simulink model "ACC_CTG_Multi_Simul"  (R2022b)
settings: Solver=VariableStepAuto  StartTime=0.0  StopTime=t_end  FixedStep=0.001  RelTol=1e-3
values from neighbouring files (symbols this model uses):
  Af = 4    [ABS_Simul_Initialize.m]    (also in ACC_CTG_Multi_Simul_Initialize.m; ACC_Space_Single_Simul_Initialize.m; ACC_Space_multi_Simul_Initialize.m; CruiseControl_Initialize.m)
  Cd = 0.3    [ABS_Simul_Initialize.m]    (also in ACC_CTG_Multi_Simul_Initialize.m; ACC_Space_Single_Simul_Initialize.m; ACC_Space_multi_Simul_Initialize.m; CruiseControl_Initialize.m)
  delta_12_0 = 600    [ACC_CTG_Multi_Simul_Initialize.m]    (also in ACC_Space_multi_Simul_Initialize.m = 550)
  delta_h1_0 = 600    [ACC_CTG_Multi_Simul_Initialize.m]    (also in ACC_Space_multi_Simul_Initialize.m = 550)
  g = 9.81    [ABS_Simul_Initialize.m]    (also in ACC_CTG_Multi_Simul_Initialize.m; ACC_Space_Single_Simul_Initialize.m; ACC_Space_multi_Simul_Initialize.m; CruiseControl_Initialize.m)
  h = 0.65    [ABS_Simul_Initialize.m]    (also in ACC_CTG_Multi_Simul_Initialize.m = 10; ACC_Space_Single_Simul_Initialize.m; ACC_Space_multi_Simul_Initialize.m; CruiseControl_Initialize.m)
  Ki_Cruise = 0.1    [ACC_CTG_Multi_Simul_Initialize.m]    (also in ACC_Space_Single_Simul_Initialize.m; ACC_Space_multi_Simul_Initialize.m)
  Kp_Cruise = 1    [ACC_CTG_Multi_Simul_Initialize.m]    (also in ACC_Space_Single_Simul_Initialize.m; ACC_Space_multi_Simul_Initialize.m)
  L_ACC = 500    [ACC_CTG_Multi_Simul_Initialize.m]    (also in ACC_Space_Single_Simul_Initialize.m; ACC_Space_multi_Simul_Initialize.m)
  lr = 1.8    [ABS_Simul_Initialize.m]    (also in ACC_CTG_Multi_Simul_Initialize.m; ACC_Space_Single_Simul_Initialize.m; ACC_Space_multi_Simul_Initialize.m; CruiseControl_Initialize.m)
  m = 1500    [ABS_Simul_Initialize.m]    (also in ACC_CTG_Multi_Simul_Initialize.m; ACC_Space_Single_Simul_Initialize.m; ACC_Space_multi_Simul_Initialize.m; CruiseControl_Initialize.m)
  ramda = 1    [ACC_CTG_Multi_Simul_Initialize.m]
  rho = 1.225    [ABS_Simul_Initialize.m]    (also in ACC_CTG_Multi_Simul_Initialize.m; ACC_Space_Single_Simul_Initialize.m; ACC_Space_multi_Simul_Initialize.m; CruiseControl_Initialize.m)
  tau = 0.5    [ACC_CTG_Multi_Simul_Initialize.m]    (also in ACC_Space_multi_Simul_Initialize.m)
  V_desire = 120    [ACC_CTG_Multi_Simul_Initialize.m]    (also in ACC_Space_Single_Simul_Initialize.m; ACC_Space_multi_Simul_Initialize.m; CruiseControl_Initialize.m = 100)
  xdot1_0 = 80    [ACC_CTG_Multi_Simul_Initialize.m]    (also in ACC_Space_multi_Simul_Initialize.m)
  xdot2_0 = 80    [ACC_CTG_Multi_Simul_Initialize.m]    (also in ACC_Space_multi_Simul_Initialize.m)
libraries: autolibshared x2, simulink x2
settings Model: Creator=lego0  LastModifiedBy=lego0

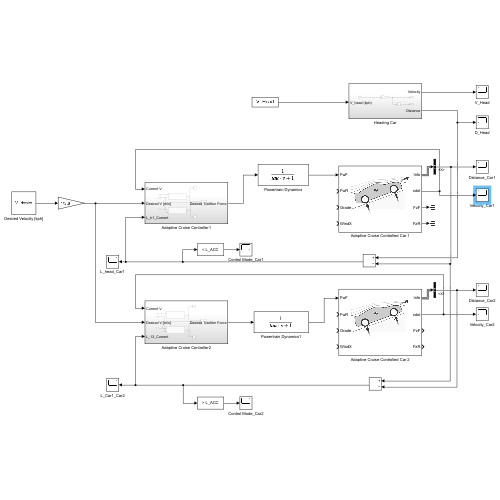
[thumbnail: Simulink's stored preview of the top-level diagram]
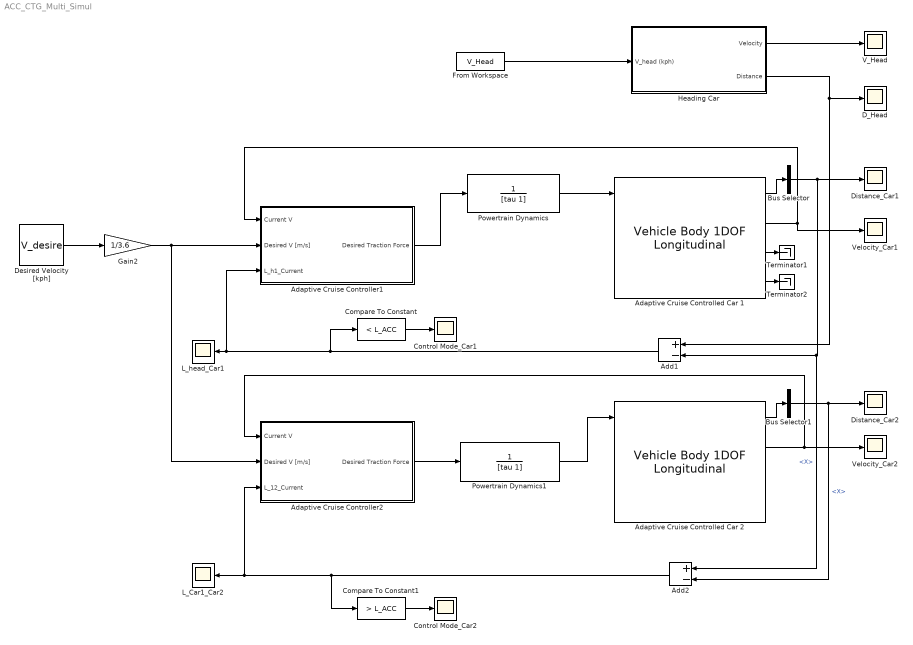
== system ACC_CTG_Multi_Simul ==
  Adaptive Cruise Controlled Car 1 : autolibshared/Vehicle Body 1DOF Longitudinal  VariantControl=SL  extFMode=off  extMMode=off  extTamb=off  wind3D=off  aMode=2  NF=2  NR=2  m=m  a=lf  b=lr  h=.35  Cd=Cd  Cl=0  Cpm=0  Af=Af  x_o=delta_12_0  xdot_o=xdot1_0/3.6  Pabs=101325  T=273  g=9.81
      settings: LibrarySourceBlock=vehdynlibeom/Vehicle Body 1DOF Longitudinal
  Adaptive Cruise Controlled Car 2 : autolibshared/Vehicle Body 1DOF Longitudinal  VariantControl=SL  extFMode=off  extMMode=off  extTamb=off  wind3D=off  aMode=2  NF=2  NR=2  m=m  a=lf  b=lr  h=.35  Cd=Cd  Cl=0  Cpm=0  Af=Af  x_o=0  xdot_o=xdot2_0/3.6  Pabs=101325  T=273  g=9.81
      settings: LibrarySourceBlock=vehdynlibeom/Vehicle Body 1DOF Longitudinal
  Adaptive Cruise Controller1 : Subsystem
  Adaptive Cruise Controller2 : Subsystem
  Add1 : Sum  Inputs=+-
  Add2 : Sum  Inputs=+-
  Bus Selector : BusSelector  OutputSignals=InertFrm.Cg.Disp.X
  Bus Selector1 : BusSelector  OutputSignals=InertFrm.Cg.Disp.X
  Compare To Constant : simulink/Logic and Bit Operations/Compare To Constant  relop=<  const=L_ACC  OutDataTypeStr=boolean
  Compare To Constant1 : simulink/Logic and Bit Operations/Compare To Constant  relop=>  const=L_ACC  OutDataTypeStr=boolean
  Control Mode_Car1 : Scope
  Control Mode_Car2 : Scope
  D_Head : Scope
  Desired Velocity [kph] : Constant  Value=V_desire
  Distance_Car1 : Scope
  Distance_Car2 : Scope
  From Workspace : FromWorkspace  VariableName=V_Head
  Gain2 : Gain  Gain=1/3.6
  Heading Car : Subsystem
  L_Car1_Car2 : Scope
  L_head_Car1 : Scope
  Powertrain Dynamics : TransferFcn  Denominator=[tau 1]
  Powertrain Dynamics1 : TransferFcn  Denominator=[tau 1]
  Terminator1 : Terminator
  Terminator2 : Terminator
  V_Head : Scope
  Velocity_Car1 : Scope
  Velocity_Car2 : Scope
  wires:
  Desired Velocity [kph]/1 -> Gain2/1
  Add1/1 -> Compare To Constant/1, L_head_Car1/1, Adaptive Cruise Controller1/3(L_h1_Current)
  Heading Car/2(Distance) -> Add1/1, D_Head/1
  From Workspace/1 -> Heading Car/1(V_head (kph))
  Heading Car/1(Velocity) -> V_Head/1
  Adaptive Cruise Controller1/1(Desired Traction Force) -> Powertrain Dynamics/1
  Gain2/1 -> Adaptive Cruise Controller2/2(Desired V [m/s]), Adaptive Cruise Controller1/2(Desired V [m/s])
  Adaptive Cruise Controller2/1(Desired Traction Force) -> Powertrain Dynamics1/1
  Add2/1 -> Compare To Constant1/1, L_Car1_Car2/1, Adaptive Cruise Controller2/3(L_12_Current)
  Powertrain Dynamics/1 -> Adaptive Cruise Controlled Car 1/1
  Adaptive Cruise Controlled Car 1/3 -> Terminator1/1
  Adaptive Cruise Controlled Car 1/4 -> Terminator2/1
  Adaptive Cruise Controlled Car 1/1 -> Bus Selector/1
  Bus Selector/1 -> Add2/1, Add1/2, Distance_Car1/1  "<X>"
  Adaptive Cruise Controlled Car 1/2 -> Velocity_Car1/1, Adaptive Cruise Controller1/1(Current V)
  Compare To Constant/1 -> Control Mode_Car1/1
  Compare To Constant1/1 -> Control Mode_Car2/1
  Powertrain Dynamics1/1 -> Adaptive Cruise Controlled Car 2/1
  Adaptive Cruise Controlled Car 2/1 -> Bus Selector1/1
  Bus Selector1/1 -> Add2/2, Distance_Car2/1  "<X>"
  Adaptive Cruise Controlled Car 2/2 -> Adaptive Cruise Controller2/1(Current V), Velocity_Car2/1

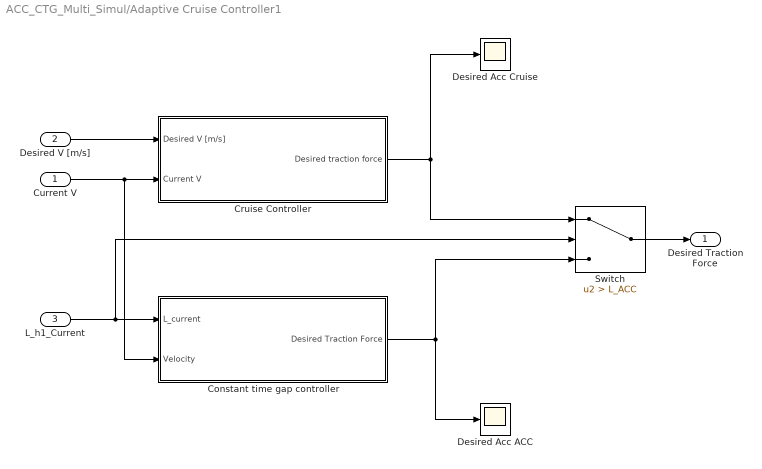
== system ACC_CTG_Multi_Simul/Adaptive Cruise Controller1 ==
  Current V : Inport
  Desired V [m/s] : Inport  Port=2
  L_h1_Current : Inport  Port=3
  Constant time gap controller : Subsystem
  Cruise Controller : Subsystem
  Desired Acc ACC : Scope
  Desired Acc Cruise : Scope
  Switch : Switch  Criteria=u2 > Threshold  Threshold=L_ACC  SaturateOnIntegerOverflow=off  InputSameDT=off
  Desired Traction Force : Outport
  wires:
  L_h1_Current/1 -> Constant time gap controller/1(L_current), Switch/2
  Constant time gap controller/1(Desired Traction Force) -> Switch/3, Desired Acc ACC/1
  Cruise Controller/1(Desired traction force) -> Desired Acc Cruise/1, Switch/1
  Desired V [m/s]/1 -> Cruise Controller/1(Desired V [m/s])
  Current V/1 -> Constant time gap controller/2(Velocity), Cruise Controller/2(Current V)
  Switch/1 -> Desired Traction Force/1

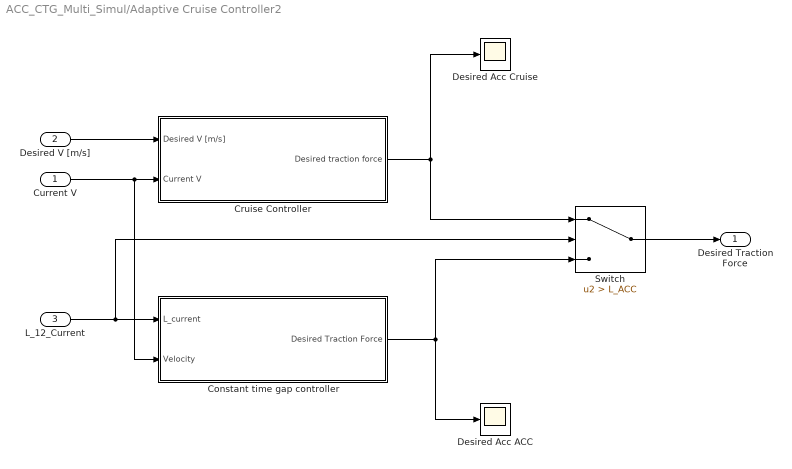
== system ACC_CTG_Multi_Simul/Adaptive Cruise Controller2 ==
  Current V : Inport
  Desired V [m/s] : Inport  Port=2
  L_12_Current : Inport  Port=3
  Constant time gap controller : Subsystem
  Cruise Controller : Subsystem
  Desired Acc ACC : Scope
  Desired Acc Cruise : Scope
  Switch : Switch  Criteria=u2 > Threshold  Threshold=L_ACC  SaturateOnIntegerOverflow=off  InputSameDT=off
  Desired Traction Force : Outport
  wires:
  L_12_Current/1 -> Constant time gap controller/1(L_current), Switch/2
  Constant time gap controller/1(Desired Traction Force) -> Switch/3, Desired Acc ACC/1
  Cruise Controller/1(Desired traction force) -> Desired Acc Cruise/1, Switch/1
  Desired V [m/s]/1 -> Cruise Controller/1(Desired V [m/s])
  Current V/1 -> Constant time gap controller/2(Velocity), Cruise Controller/2(Current V)
  Switch/1 -> Desired Traction Force/1

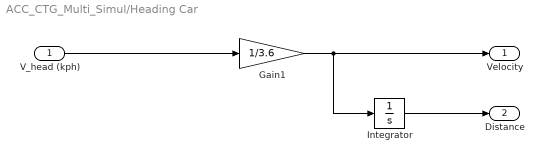
== system ACC_CTG_Multi_Simul/Heading Car ==
  V_head (kph) : Inport
  Gain1 : Gain  Gain=1/3.6
  Integrator : Integrator  InitialCondition=delta_h1_0 + delta_12_0
  Velocity : Outport
  Distance : Outport  Port=2
  wires:
  Gain1/1 -> Velocity/1, Integrator/1
  Integrator/1 -> Distance/1
  V_head (kph)/1 -> Gain1/1

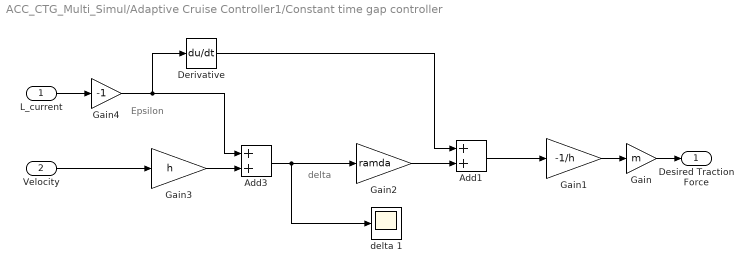
== system ACC_CTG_Multi_Simul/Adaptive Cruise Controller1/Constant time gap controller ==
  note: delta
  note: Epsilon
  L_current : Inport
  Velocity : Inport  Port=2
  Add1 : Sum
  Add3 : Sum
  Derivative : Derivative
  Gain : Gain  Gain=m
  Gain1 : Gain  Gain=-1/h
  Gain2 : Gain  Gain=ramda
  Gain3 : Gain  Gain=h
  Gain4 : Gain  Gain=-1
  delta 1 : Scope
  Desired Traction Force : Outport
  wires:
  Velocity/1 -> Gain3/1
  Gain3/1 -> Add3/2
  Add3/1 -> delta 1/1, Gain2/1
  L_current/1 -> Gain4/1
  Gain4/1 -> Derivative/1, Add3/1
  Gain2/1 -> Add1/2
  Derivative/1 -> Add1/1
  Add1/1 -> Gain1/1
  Gain1/1 -> Gain/1
  Gain/1 -> Desired Traction Force/1

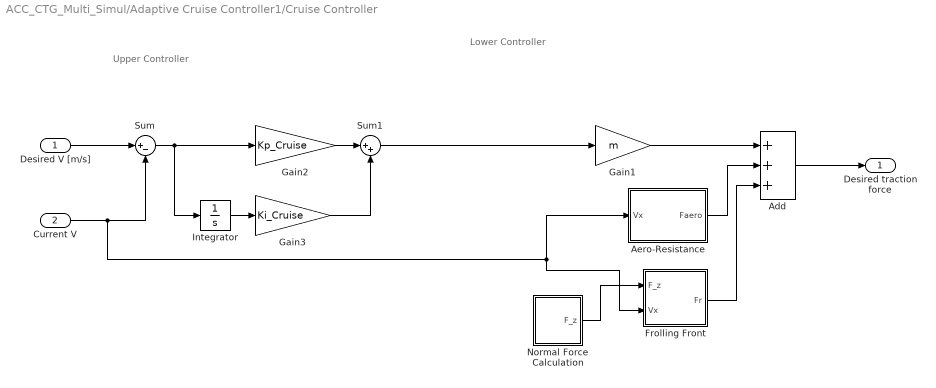
== system ACC_CTG_Multi_Simul/Adaptive Cruise Controller1/Cruise Controller ==
  note: Upper Controller
  note: Lower Controller
  Desired V [m/s] : Inport
  Current V : Inport  Port=2
  Add : Sum  Inputs=+++
  Aero-Resistance : Subsystem
  Frolling Front : Subsystem
  Gain1 : Gain  Gain=m
  Gain2 : Gain  Gain=Kp_Cruise
  Gain3 : Gain  Gain=Ki_Cruise
  Integrator : Integrator
  Normal Force Calculation : Subsystem
  Sum : Sum  Inputs=|+-
  Sum1 : Sum  Inputs=|++
  Desired traction force : Outport
  wires:
  Gain2/1 -> Sum1/1
  Current V/1 -> Frolling Front/2(Vx), Aero-Resistance/1(Vx), Sum/2
  Gain3/1 -> Sum1/2
  Sum/1 -> Integrator/1, Gain2/1
  Integrator/1 -> Gain3/1
  Desired V [m/s]/1 -> Sum/1
  Sum1/1 -> Gain1/1
  Gain1/1 -> Add/1
  Add/1 -> Desired traction force/1
  Normal Force Calculation/1(F_z) -> Frolling Front/1(F_z)
  Aero-Resistance/1(Faero) -> Add/2
  Frolling Front/1(Fr) -> Add/3

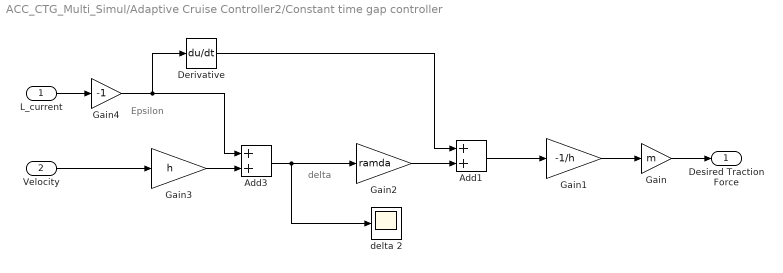
== system ACC_CTG_Multi_Simul/Adaptive Cruise Controller2/Constant time gap controller ==
  note: delta
  note: Epsilon
  L_current : Inport
  Velocity : Inport  Port=2
  Add1 : Sum
  Add3 : Sum
  Derivative : Derivative
  Gain : Gain  Gain=m
  Gain1 : Gain  Gain=-1/h
  Gain2 : Gain  Gain=ramda
  Gain3 : Gain  Gain=h
  Gain4 : Gain  Gain=-1
  delta 2 : Scope
  Desired Traction Force : Outport
  wires:
  Velocity/1 -> Gain3/1
  Gain3/1 -> Add3/2
  Add3/1 -> delta 2/1, Gain2/1
  L_current/1 -> Gain4/1
  Gain4/1 -> Derivative/1, Add3/1
  Gain2/1 -> Add1/2
  Derivative/1 -> Add1/1
  Add1/1 -> Gain1/1
  Gain1/1 -> Gain/1
  Gain/1 -> Desired Traction Force/1

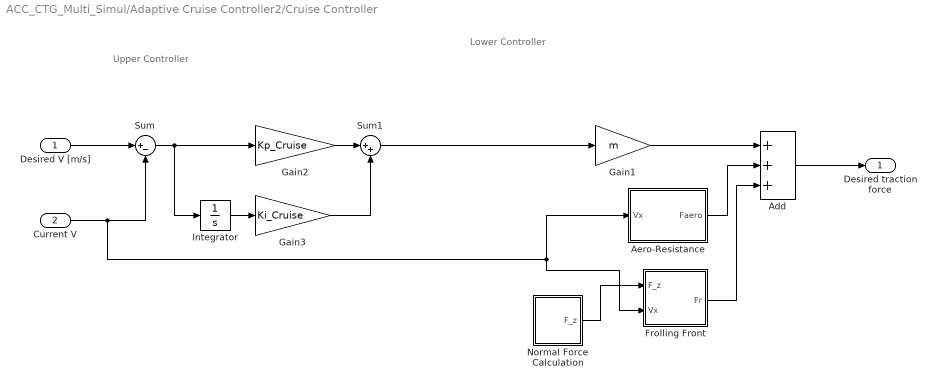
== system ACC_CTG_Multi_Simul/Adaptive Cruise Controller2/Cruise Controller ==
  note: Upper Controller
  note: Lower Controller
  Desired V [m/s] : Inport
  Current V : Inport  Port=2
  Add : Sum  Inputs=+++
  Aero-Resistance : Subsystem
  Frolling Front : Subsystem
  Gain1 : Gain  Gain=m
  Gain2 : Gain  Gain=Kp_Cruise
  Gain3 : Gain  Gain=Ki_Cruise
  Integrator : Integrator
  Normal Force Calculation : Subsystem
  Sum : Sum  Inputs=|+-
  Sum1 : Sum  Inputs=|++
  Desired traction force : Outport
  wires:
  Gain2/1 -> Sum1/1
  Current V/1 -> Frolling Front/2(Vx), Aero-Resistance/1(Vx), Sum/2
  Gain3/1 -> Sum1/2
  Sum/1 -> Integrator/1, Gain2/1
  Integrator/1 -> Gain3/1
  Desired V [m/s]/1 -> Sum/1
  Sum1/1 -> Gain1/1
  Gain1/1 -> Add/1
  Add/1 -> Desired traction force/1
  Normal Force Calculation/1(F_z) -> Frolling Front/1(F_z)
  Aero-Resistance/1(Faero) -> Add/2
  Frolling Front/1(Fr) -> Add/3

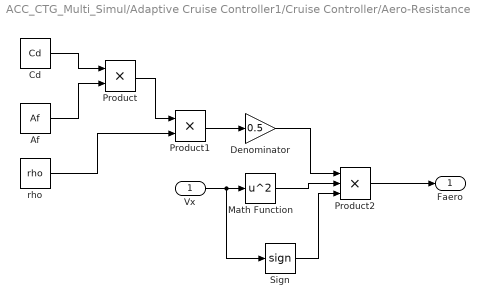
== system ACC_CTG_Multi_Simul/Adaptive Cruise Controller1/Cruise Controller/Aero-Resistance ==
  Vx : Inport
  Af : Constant  Value=Af
  Cd : Constant  Value=Cd
  Denominator : Gain  Gain=0.5
  Math Function : Math  Operator=square  SignedPower=on
  Product : Product
  Product1 : Product
  Product2 : Product  Inputs=3
  Sign : Signum
  rho : Constant  Value=rho
  Faero : Outport  VectorParamsAs1DForOutWhenUnconnected=off
  wires:
  Af/1 -> Product/2
  Product1/1 -> Denominator/1
  Denominator/1 -> Product2/1
  Vx/1 -> Sign/1, Math Function/1
  rho/1 -> Product1/2
  Cd/1 -> Product/1
  Math Function/1 -> Product2/2
  Product/1 -> Product1/1
  Sign/1 -> Product2/3
  Product2/1 -> Faero/1

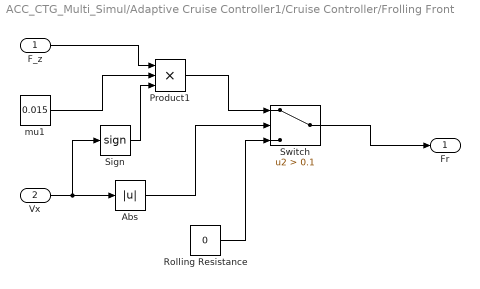
== system ACC_CTG_Multi_Simul/Adaptive Cruise Controller1/Cruise Controller/Frolling Front ==
  F_z : Inport
  Vx : Inport  Port=2
  Abs : Abs  SaturateOnIntegerOverflow=off
  Product1 : Product  Inputs=3
  Rolling Resistance : Constant  Value=0
  Sign : Signum
  Switch : Switch  Criteria=u2 > Threshold  Threshold=0.1  SaturateOnIntegerOverflow=off  InputSameDT=off
  mu1 : Constant  Value=0.015
  Fr : Outport  VectorParamsAs1DForOutWhenUnconnected=off
  wires:
  F_z/1 -> Product1/1
  Product1/1 -> Switch/1
  Rolling Resistance/1 -> Switch/3
  mu1/1 -> Product1/2
  Vx/1 -> Sign/1, Abs/1
  Abs/1 -> Switch/2
  Sign/1 -> Product1/3
  Switch/1 -> Fr/1

== system ACC_CTG_Multi_Simul/Adaptive Cruise Controller1/Cruise Controller/Normal Force Calculation ==
  Constant : Constant  Value=m
  Constant1 : Constant  Value=g
  Product : Product
  F_z : Outport
  wires:
  Product/1 -> F_z/1
  Constant1/1 -> Product/2
  Constant/1 -> Product/1

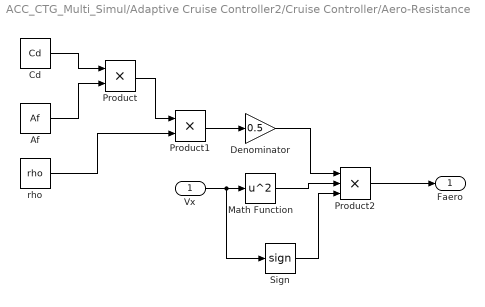
== system ACC_CTG_Multi_Simul/Adaptive Cruise Controller2/Cruise Controller/Aero-Resistance ==
  Vx : Inport
  Af : Constant  Value=Af
  Cd : Constant  Value=Cd
  Denominator : Gain  Gain=0.5
  Math Function : Math  Operator=square  SignedPower=on
  Product : Product
  Product1 : Product
  Product2 : Product  Inputs=3
  Sign : Signum
  rho : Constant  Value=rho
  Faero : Outport  VectorParamsAs1DForOutWhenUnconnected=off
  wires:
  Af/1 -> Product/2
  Product1/1 -> Denominator/1
  Denominator/1 -> Product2/1
  Vx/1 -> Sign/1, Math Function/1
  rho/1 -> Product1/2
  Cd/1 -> Product/1
  Math Function/1 -> Product2/2
  Product/1 -> Product1/1
  Sign/1 -> Product2/3
  Product2/1 -> Faero/1

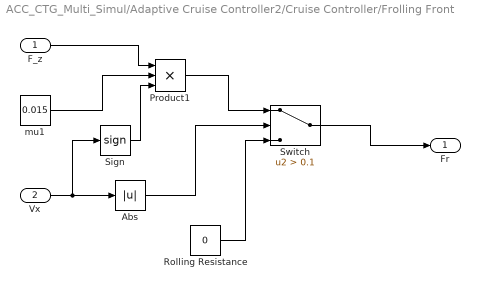
== system ACC_CTG_Multi_Simul/Adaptive Cruise Controller2/Cruise Controller/Frolling Front ==
  F_z : Inport
  Vx : Inport  Port=2
  Abs : Abs  SaturateOnIntegerOverflow=off
  Product1 : Product  Inputs=3
  Rolling Resistance : Constant  Value=0
  Sign : Signum
  Switch : Switch  Criteria=u2 > Threshold  Threshold=0.1  SaturateOnIntegerOverflow=off  InputSameDT=off
  mu1 : Constant  Value=0.015
  Fr : Outport  VectorParamsAs1DForOutWhenUnconnected=off
  wires:
  F_z/1 -> Product1/1
  Product1/1 -> Switch/1
  Rolling Resistance/1 -> Switch/3
  mu1/1 -> Product1/2
  Vx/1 -> Sign/1, Abs/1
  Abs/1 -> Switch/2
  Sign/1 -> Product1/3
  Switch/1 -> Fr/1

== system ACC_CTG_Multi_Simul/Adaptive Cruise Controller2/Cruise Controller/Normal Force Calculation ==
  Constant : Constant  Value=m
  Constant1 : Constant  Value=g
  Product : Product
  F_z : Outport
  wires:
  Product/1 -> F_z/1
  Constant1/1 -> Product/2
  Constant/1 -> Product/1
